simulink model "rc_ckt_Model"  (R2020a)
settings: Solver=VariableStepAuto  StartTime=0.0  StopTime=10.0  RelTol=1e-3
settings Model: Creator=INDRAJIT MARATHE  LastModifiedBy=INDRAJIT MARATHE

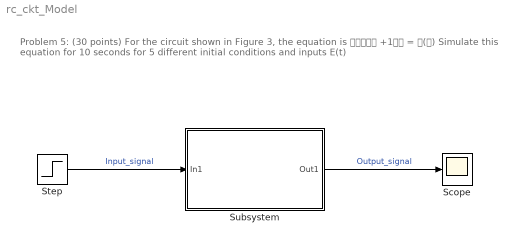
== system rc_ckt_Model ==
  note: Problem 5: (30 points) For the circuit shown in Figure 3, the equation is
      | 𝑅𝑑𝑄𝑑𝑡 +1𝐶𝑄 = 𝐸(𝑡)
      | Simulate this equation for 10 seconds for 5 different initial conditions and inputs E(t)
  Scope : Scope
  Step : Step  Time=2  SampleTime=0
  Subsystem : Subsystem
  wires:
  Step/1 -> Subsystem/1(In1)  "Input_signal"
  Subsystem/1(Out1) -> Scope/1  "Output_signal"

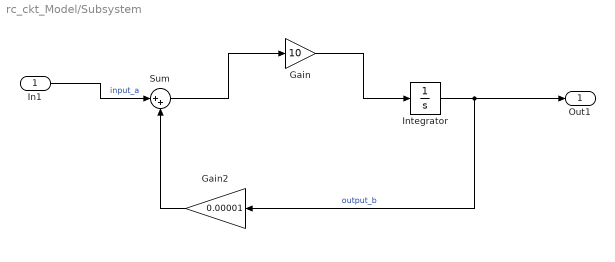
== system rc_ckt_Model/Subsystem ==
  In1 : Inport
  Gain : Gain  Gain=10
  Gain2 : Gain  Gain=0.00001
  Integrator : Integrator
  Sum : Sum  Inputs=|++
  Out1 : Outport
  wires:
  Sum/1 -> Gain/1
  In1/1 -> Sum/1  "input_a"
  Integrator/1 -> Gain2/1, Out1/1  "output_b"
  Gain2/1 -> Sum/2
  Gain/1 -> Integrator/1
